simulink model "heading_autopilot_PIDcontrol"  (R2022a)
settings: Solver=VariableStepAuto  StartTime=0.0  StopTime=10.0  RelTol=1e-3
values from neighbouring files (symbols this model uses):
  T = [1 0 0.075 1 0 -0.075 0 1 0.465 0 1 -0.595 ... (15 elements, 3x5)]    [CompleteTest.mat]    (also in NoHeading.mat; statefeedback.mat = 77000)
libraries: mssSimulink x1
settings Model: Creator=XinyiWu  LastModifiedBy=XinyiWu

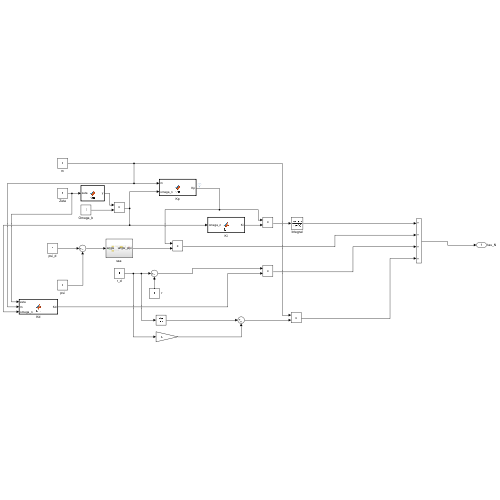
[thumbnail: Simulink's stored preview of the top-level diagram]
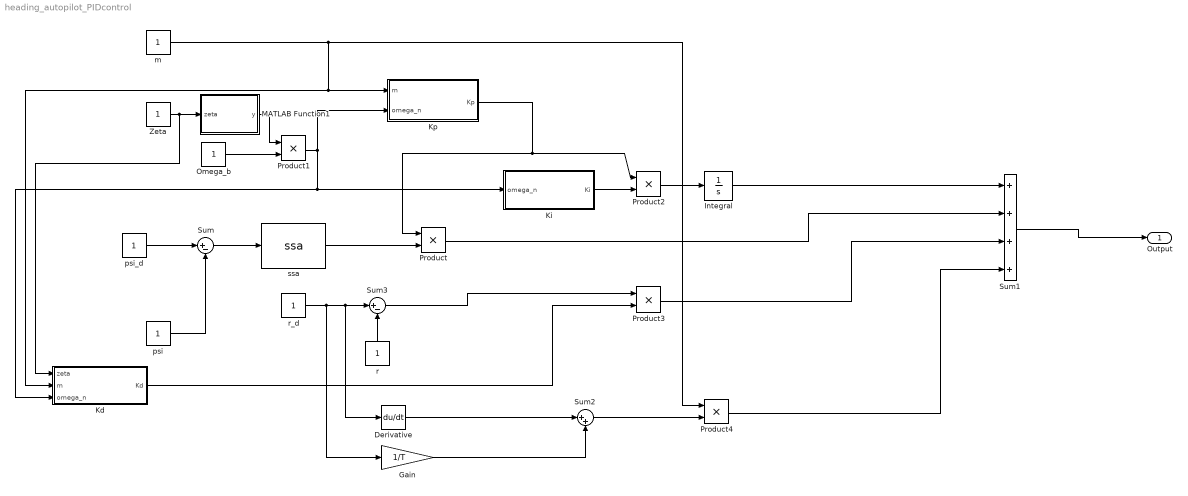
== system heading_autopilot_PIDcontrol ==
  Derivative : Derivative
  Gain : Gain  Gain=1/T
  Integral : TransferFcn  Denominator=[1 0]
  Kd : MATLAB Function  TreatAsAtomicUnit=on
  Ki : MATLAB Function  TreatAsAtomicUnit=on
  Kp : MATLAB Function  TreatAsAtomicUnit=on
  MATLAB Function1 : MATLAB Function  TreatAsAtomicUnit=on
  Omega_b : Constant
  Product{,1..4} (5 alike) : Product
  Sum : Sum  Inputs=|+-
  Sum1 : Sum  Inputs=++++  InputSameDT=on  SaturateOnIntegerOverflow=on  OutDataTypeStr=Inherit: Same as first input
  Sum2 : Sum  Inputs=|++
  Sum3 : Sum  Inputs=|+-  InputSameDT=on  SaturateOnIntegerOverflow=on  OutDataTypeStr=Inherit: Same as first input
  Zeta : Constant
  m : Constant
  psi : Constant
  psi_d : Constant
  r : Constant
  r_d : Constant
  "ssa " : mssSimulink/Utilities/Math Operations/ssa  SystemSampleTime=-1  VariantActivationTime=update diagram  Latency=0  AutoFrameSizeCalculation=off
  Output : Outport  SignalName=tau_N
  wires:
  Sum1/1 -> Output/1
  Product3/1 -> Sum1/3
  Product2/1 -> Integral/1
  "ssa "/1 -> Product/2
  Sum3/1 -> Product3/1
  r/1 -> Sum3/2
  psi_d/1 -> Sum/1
  Sum/1 -> "ssa "/1
  r_d/1 -> Gain/1, Derivative/1, Sum3/1
  psi/1 -> Sum/2
  MATLAB Function1/1(y) -> Product1/1
  Omega_b/1 -> Product1/2
  Product1/1 -> Kd/3(omega_n), Ki/1(omega_n), Kp/2(omega_n)
  Zeta/1 -> Kd/1(zeta), MATLAB Function1/1(zeta)
  Kp/1(Kp) -> Product2/1, Product/1
  Ki/1(Ki) -> Product2/2
  Kd/1(Kd) -> Product3/2
  m/1 -> Kd/2(m), Kp/1(m), Product4/1
  Derivative/1 -> Sum2/1
  Gain/1 -> Sum2/2
  Sum2/1 -> Product4/2
  Product4/1 -> Sum1/4
  Product/1 -> Sum1/2
  Integral/1 -> Sum1/1

== matlab function heading_autopilot_PIDcontrol/Kp ==
  data: m input; omega_n input; Kp output
function Kp   = fcn(m, omega_n)

Kp = m*(omega_n)^2;

== matlab function heading_autopilot_PIDcontrol/Ki ==
  data: omega_n input; Ki output
function Ki = fcn(omega_n)

Ki = (omega_n)/10;

== matlab function heading_autopilot_PIDcontrol/Kd ==
  data: zeta input; m input; omega_n input; Kd output
function Kd = fcn(zeta, m, omega_n)

Kd = 2*zeta*omega_n*m;

== matlab function heading_autopilot_PIDcontrol/MATLAB Function1 ==
  data: zeta input; y output
function y = fcn(zeta)

y = 1/sqrt((1-2*zeta^2)+sqrt(4*zeta^4-4*zeta^2+2));
